simulink model "OperationalSpaceGravityCompensation"  (R2021a)
settings: Solver=ode4  StartTime=0.0  StopTime=3  FixedStep=0.001  RelTol=1e-3
values from neighbouring files (symbols this model uses):
  kd = diag([50 30 10 10 10 10])    [params.m]
  kp = diag([250 200 150 30 30 50])    [params.m]
  x = [pose' , or']'    [compute_custom_pose.m]    (also in params.m = [ 0.5357)
settings Model: Creator=Sebastiano  LastModifiedBy=antoninoparisi
settings SolverCC: AlgebraicLoopSolver=TrustRegion
settings DebuggingCC: SFMachineParentedDataDiag=warning

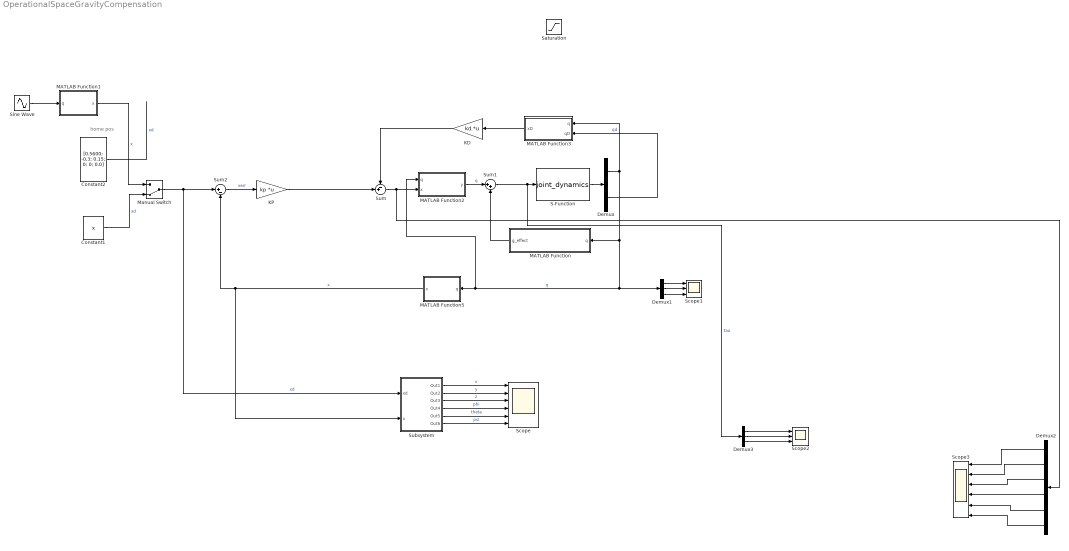
== system OperationalSpaceGravityCompensation ==
  note: home pos
  Constant1 : Constant  Value=x  VectorParams1D=off
  Constant2 : Constant  Value=[0.5600; -0.3; 0.15; 0; 0; 0.0]  VectorParams1D=off
  Demux : Demux  Outputs=[3, 3]
  Demux1 : Demux  Outputs=3
  Demux2 : Demux  Outputs=6
  Demux3 : Demux  Outputs=3
  KD : Gain  Gain=kd  Multiplication=Matrix(K*u) (u vector)
  KP : Gain  Gain=kp  Multiplication=Matrix(K*u) (u vector)
  MATLAB Function : MATLAB Function  TreatAsAtomicUnit=on
  MATLAB Function1 : MATLAB Function  TreatAsAtomicUnit=on
  MATLAB Function2 : MATLAB Function  TreatAsAtomicUnit=on
  MATLAB Function3 : MATLAB Function  TreatAsAtomicUnit=on
  MATLAB Function5 : MATLAB Function  TreatAsAtomicUnit=on
  Manual Switch : ManualSwitch  CurrentSetting=0
  S-Function : S-Function  FunctionName=joint_dynamics  Parameters=robot  SFunctionDeploymentMode=off  EnableBusSupport=off
  Saturation : Saturate  UpperLimit=500  LowerLimit=-500
  Scope : Scope  NumInputPorts=6
  Scope1 : Scope  NumInputPorts=3
  Scope2 : Scope  NumInputPorts=3
  Scope3 : Scope  NumInputPorts=6
  Sine Wave : Sin  Amplitude=0.05  SampleTime=0
  Subsystem : Subsystem
  Sum : Sum  Inputs=-+|
  Sum1 : Sum  Inputs=|++
  Sum2 : Sum  Inputs=|+-
  wires:
  KP/1 -> Sum/2
  Sum2/1 -> KP/1  "xerr"
  MATLAB Function/1(g_effect) -> Sum1/2
  S-Function/1 -> Demux/1
  Sum1/1 -> Demux3/1, S-Function/1  "tau"
  Sum/1 -> Demux2/1, MATLAB Function2/2(x)
  KD/1 -> Sum/1
  MATLAB Function5/1(x) -> Subsystem/2(x), Sum2/2  "x"
  MATLAB Function3/1(xD) -> KD/1
  Manual Switch/1 -> Subsystem/1(xd), Sum2/1  "xd"
  Constant1/1 -> Manual Switch/2  "xd"
  Constant2/1 -> ?  "xd"
  Subsystem/1(Out1) -> Scope/1  "x"
  Subsystem/2(Out2) -> Scope/2  "y"
  Subsystem/3(Out3) -> Scope/3  "z"
  Subsystem/4(Out4) -> Scope/4  "phi"
  Subsystem/5(Out5) -> Scope/5  "theta"
  Subsystem/6(Out6) -> Scope/6  "psi"
  Demux/1 -> Demux1/1, MATLAB Function2/1(q), MATLAB Function5/1(q), MATLAB Function/1(q), MATLAB Function3/1(q)  "q"
  Demux/2 -> MATLAB Function3/2(qD)  "qd"
  Demux1/1 -> Scope1/1
  Demux1/2 -> Scope1/2
  Demux1/3 -> Scope1/3
  MATLAB Function2/1(y) -> Sum1/1  "q"
  Demux2/1 -> Scope3/1
  Demux2/2 -> Scope3/2
  Demux2/3 -> Scope3/3
  Demux2/4 -> Scope3/4
  Demux2/5 -> Scope3/5
  Demux2/6 -> Scope3/6
  Demux3/2 -> Scope2/2
  Demux3/1 -> Scope2/1
  Demux3/3 -> Scope2/3
  Sine Wave/1 -> MATLAB Function1/1(q)
  MATLAB Function1/1(x) -> Manual Switch/1  "x"

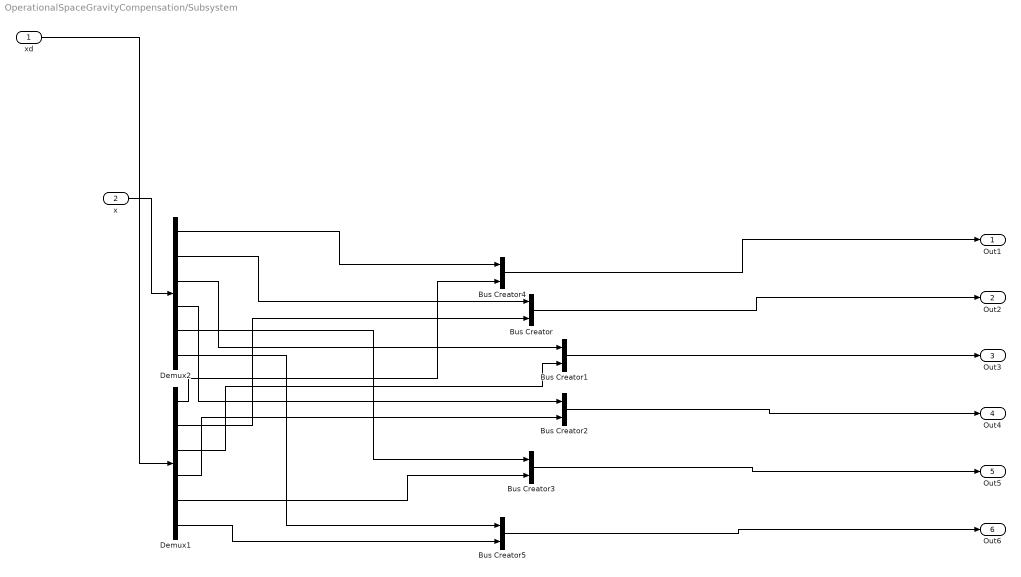
== system OperationalSpaceGravityCompensation/Subsystem ==
  xd : Inport
  x : Inport  Port=2
  Bus Creator{,1..5} (6 alike) : BusCreator  Inputs=2
  Demux1 : Demux  Outputs=6
  Demux2 : Demux  Outputs=6
  Out1 : Outport
  Out2 : Outport  Port=2
  Out3 : Outport  Port=3
  Out4 : Outport  Port=4
  Out5 : Outport  Port=5
  Out6 : Outport  Port=6
  wires:
  xd/1 -> Demux1/1
  x/1 -> Demux2/1
  Bus Creator1/1 -> Out3/1
  Bus Creator4/1 -> Out1/1
  Demux2/2 -> Bus Creator/1
  Demux1/1 -> Bus Creator4/2
  Demux1/3 -> Bus Creator1/2
  Demux2/3 -> Bus Creator1/1
  Demux2/6 -> Bus Creator5/1
  Demux2/4 -> Bus Creator2/1
  Bus Creator5/1 -> Out6/1
  Demux2/1 -> Bus Creator4/1
  Bus Creator/1 -> Out2/1
  Demux1/6 -> Bus Creator5/2
  Demux1/2 -> Bus Creator/2
  Demux1/5 -> Bus Creator3/2
  Bus Creator2/1 -> Out4/1
  Demux1/4 -> Bus Creator2/2
  Bus Creator3/1 -> Out5/1
  Demux2/5 -> Bus Creator3/1

== matlab function OperationalSpaceGravityCompensation/MATLAB Function ==
  data: q input; g_effect output
function g_effect = gravity(q)

g_effect = G_Lagrangian(q);

== matlab function OperationalSpaceGravityCompensation/MATLAB Function2 ==
  data: q input; y output size=3; x input
function y = JAT(q, x)

y = analyticalJacobian(q)' * x;

== matlab function OperationalSpaceGravityCompensation/MATLAB Function3 ==
  data: q input; xD output size=6; qD input
function xD = JA(q, qD)

xD = analyticalJacobian(q)*qD;

== matlab function OperationalSpaceGravityCompensation/MATLAB Function5 ==
  data: q input; x output
function x = K(q)

t1 = q(1);
d1 = q(2);
t2 = q(3);


a1 = 0.15;
a2 = 0.4;
a3 = 0.3;
a4 = 0.16;


% wrt frame 0
K = [[cos(t1)*cos(t2), -cos(t1)*sin(t2), -sin(t1),      a2*cos(t1) + a4*cos(t1)*cos(t2)]
    [        sin(t2),          cos(t2),        0,                 a4*sin(t2) - d1 - a3]
    [cos(t2)*sin(t1), -sin(t1)*sin(t2),  cos(t1), a1 + a2*sin(t1) + a4*cos(t2)*sin(t1)]
    [              0,                0,        0,                                    1]];

pos = K(1:3, 4);
ori = rotm2eul(K(1:3,1:3), 'ZYZ')';

x = [pos; ori];

== matlab function OperationalSpaceGravityCompensation/MATLAB Function1 ==
  data: q input; x output
function x = K(q)

t1 = q;
d1 = q;
t2 = q;


a1 = 0.15;
a2 = 0.4;
a3 = 0.3;
a4 = 0.16;


% wrt frame 0
K = [[cos(t1)*cos(t2), -cos(t1)*sin(t2), -sin(t1),      a2*cos(t1) + a4*cos(t1)*cos(t2)]
    [        sin(t2),          cos(t2),        0,                 a4*sin(t2) - d1 - a3]
    [cos(t2)*sin(t1), -sin(t1)*sin(t2),  cos(t1), a1 + a2*sin(t1) + a4*cos(t2)*sin(t1)]
    [              0,                0,        0,                                    1]];

pos = K(1:3, 4);
ori = rotm2eul(K(1:3,1:3), 'ZYZ')';

x = [pos; ori];
